simulink model "systemWithController"  (R2020a)
settings: Solver=VariableStepAuto  StartTime=0.0  StopTime=10.0  RelTol=1e-3
InitFcn:
  | modelParam
values from neighbouring files (symbols this model uses):
  Kd = K*T    [Untitled2.m]    (also in modelParam.m; widePosSysAnal.m)
  Ki = 10    [widePosSysAnal.m]
  Kp = K*Zc/Pc    [Untitled2.m]    (also in modelParam.m; widePosSysAnal.m)
undefined symbols (not defined in the file or in its folder): gpden, gpnum
settings Model: Creator=tumma  LastModifiedBy=tumma
settings DataIOCC: ReturnWorkspaceOutputs=off
settings DebuggingCC: ArithmeticOperatorsInVariantConditions=warning
settings SFSimCC: SimUseLocalCustomCode=off  CustomCodeUndefinedFunction=UseInterfaceOnly
settings RTWCC: RTWUseLocalCustomCode=off

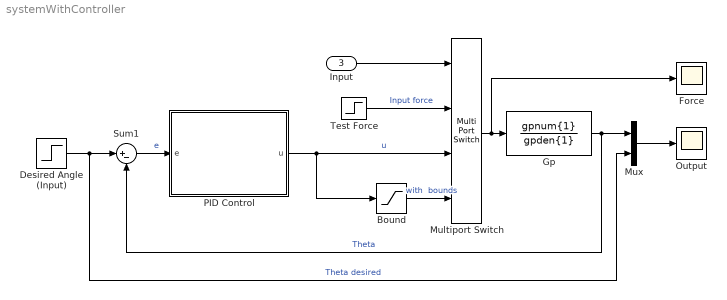
== system systemWithController ==
  Input : Inport  Port=3
  "Bound " : Saturate  UpperLimit=0.411  LowerLimit=0
  Desired Angle (Input) : Step  After=15  SampleTime=0
  Force : Scope
  Gp : TransferFcn  Numerator=gpnum{1}  Denominator=gpden{1}
  Multiport Switch : MultiPortSwitch
  Mux : Mux  Inputs=2
  "Output " : Scope
  PID Control : Subsystem
  Sum1 : Sum  Inputs=|+-
  Test Force : Step  After=0.0901  SampleTime=0
  wires:
  Test Force/1 -> Multiport Switch/2  "Input force"
  Gp/1 -> Mux/1, Sum1/2  "Theta"
  Multiport Switch/1 -> Force/1, Gp/1
  Desired Angle (Input)/1 -> Sum1/1, Mux/2  "Theta desired"
  "Bound "/1 -> Multiport Switch/4  "with  bounds"
  Mux/1 -> "Output "/1
  Input/1 -> Multiport Switch/1
  PID Control/1(u) -> "Bound "/1, Multiport Switch/3  "u"
  Sum1/1 -> PID Control/1(e)  "e"

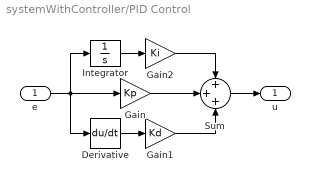
== system systemWithController/PID Control ==
  e : Inport
  Derivative : Derivative
  Gain : Gain  Gain=Kp
  Gain1 : Gain  Gain=Kd
  Gain2 : Gain  Gain=Ki
  Integrator : Integrator
  Sum : Sum  Inputs=+++
  u : Outport
  wires:
  Derivative/1 -> Gain1/1
  Gain1/1 -> Sum/3
  e/1 -> Integrator/1, Derivative/1, Gain/1
  Sum/1 -> u/1
  Gain/1 -> Sum/2
  Integrator/1 -> Gain2/1
  Gain2/1 -> Sum/1
